simulink model "adaptive_try2"  (R2020a)
settings: Solver=VariableStepAuto  StartTime=0.0  StopTime=10.0  RelTol=1e-3
libraries: powerlib_meascontrol x6
settings Model: Creator=sulai  LastModifiedBy=sulai

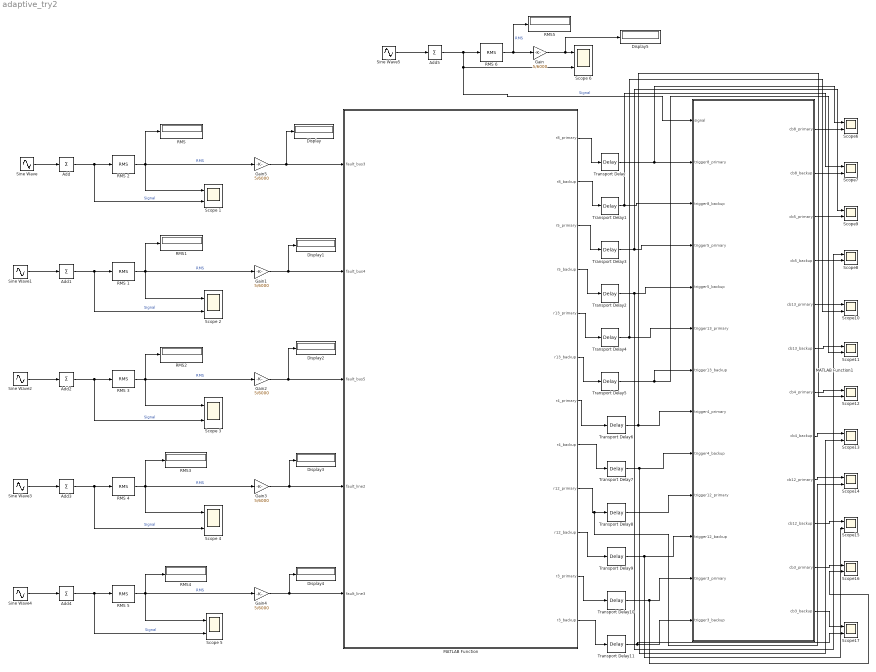
== system adaptive_try2 ==
  Add{,1..5} (6 alike) : Sum  Inputs=+  SampleTime=0
  Display{,1..5} (6 alike) : Display
  Gain{,1..5} (6 alike) : Gain  Gain=5/6000
  MATLAB Function : MATLAB Function  TreatAsAtomicUnit=on
  MATLAB Function1 : MATLAB Function  TreatAsAtomicUnit=on
  RMS{,1..5} (6 alike) : Display
      settings: Format=bank
  RMS {1..4} (4 alike) : powerlib_meascontrol/Measurements/RMS  TrueRMS=off  Freq=60  RMSInit=120  Ts=0
  RMS 5 : powerlib_meascontrol/Measurements/RMS  TrueRMS=off  Freq=10  RMSInit=120  Ts=0
  RMS 6 : powerlib_meascontrol/Measurements/RMS  TrueRMS=off  Freq=10  RMSInit=120  Ts=0
  Scope {1..6} (6 alike) : Scope  NumInputPorts=2
  Scope{6..17} (12 alike) : Scope  NumInputPorts=2
  Sine Wave{,1..3} (4 alike) : Sin  Amplitude=2  Frequency=2*pi*60  SampleTime=0
  Sine Wave4 : Sin  Amplitude=9000  Frequency=2*pi*10  SampleTime=0
  Sine Wave5 : Sin  Amplitude=126000  Frequency=2*pi*10  SampleTime=0
  Transport Delay{,3..4,6,8,10} (6 alike) : TransportDelay  DelayTime=0.2
  Transport Delay{1..2,5,7,9,11} (6 alike) : TransportDelay  DelayTime=1.86
  wires:
  MATLAB Function/2(r8_backup) -> Transport Delay1/1
  MATLAB Function/3(r5_primary) -> Transport Delay3/1
  MATLAB Function/4(r5_backup) -> Transport Delay2/1
  MATLAB Function/5(r13_primary) -> Transport Delay4/1
  MATLAB Function/6(r13_backup) -> Transport Delay5/1
  MATLAB Function/7(r4_primary) -> Transport Delay6/1
  MATLAB Function/8(r4_backup) -> Transport Delay7/1
  MATLAB Function/9(r12_primary) -> Scope14/2, Transport Delay8/1
  MATLAB Function/11(r3_primary) -> Transport Delay10/1
  MATLAB Function/12(r3_backup) -> Transport Delay11/1
  MATLAB Function/1(r8_primary) -> Transport Delay/1
  MATLAB Function/10(r12_backup) -> Transport Delay9/1
  Transport Delay9/1 -> Scope15/2, MATLAB Function1/11(trigger12_backup)
  Transport Delay8/1 -> MATLAB Function1/10(trigger12_primary)
  Transport Delay7/1 -> Scope13/2, MATLAB Function1/9(trigger4_backup)
  Transport Delay6/1 -> Scope12/2, MATLAB Function1/8(trigger4_primary)
  Transport Delay5/1 -> Scope11/2, MATLAB Function1/7(trigger13_backup)
  Transport Delay4/1 -> Scope10/2, MATLAB Function1/6(trigger13_primary)
  Transport Delay2/1 -> Scope8/1, MATLAB Function1/5(trigger5_backup)
  Transport Delay3/1 -> Scope9/1, MATLAB Function1/4(trigger5_primary)
  Transport Delay1/1 -> Scope7/1, MATLAB Function1/3(trigger8_backup)
  Transport Delay/1 -> Scope6/1, MATLAB Function1/2(trigger8_primary)
  MATLAB Function1/1(cb8_primary) -> Scope6/2
  MATLAB Function1/2(cb8_backup) -> Scope7/2
  MATLAB Function1/3(cb5_primary) -> Scope9/2
  MATLAB Function1/4(cb5_backup) -> Scope8/2
  MATLAB Function1/5(cb13_primary) -> Scope10/1
  MATLAB Function1/6(cb13_backup) -> Scope11/1
  MATLAB Function1/7(cb4_primary) -> Scope12/1
  MATLAB Function1/8(cb4_backup) -> Scope13/1
  MATLAB Function1/9(cb12_primary) -> Scope14/1
  MATLAB Function1/10(cb12_backup) -> Scope15/1
  MATLAB Function1/11(cb3_primary) -> Scope16/1
  MATLAB Function1/12(cb3_backup) -> Scope17/1
  Transport Delay10/1 -> Scope16/2, MATLAB Function1/12(trigger3_primary)
  Transport Delay11/1 -> Scope17/2, MATLAB Function1/13(trigger3_backup)
  Sine Wave/1 -> Add/1
  RMS 2/1 -> Scope 1/1, RMS/1, Gain5/1  "RMS"
  Add/1 -> Scope 1/2, RMS 2/1  "Signal"
  Gain5/1 -> Display/1, MATLAB Function/1(fault_bus3)
  Gain1/1 -> Display1/1, MATLAB Function/2(fault_bus4)
  Add1/1 -> Scope 2/2, RMS 1/1  "Signal"
  RMS 1/1 -> Scope 2/1, RMS1/1, Gain1/1  "RMS"
  Sine Wave1/1 -> Add1/1
  Gain2/1 -> Display2/1, MATLAB Function/3(fault_bus5)
  Add2/1 -> Scope 3/2, RMS 3/1  "Signal"
  RMS 3/1 -> Scope 3/1, RMS2/1, Gain2/1  "RMS"
  Sine Wave2/1 -> Add2/1
  Gain3/1 -> Display3/1, MATLAB Function/4(fault_line2)
  Add3/1 -> Scope 4/2, RMS 4/1  "Signal"
  RMS 4/1 -> Scope 4/1, RMS3/1, Gain3/1  "RMS"
  Sine Wave3/1 -> Add3/1
  Gain4/1 -> Display4/1, MATLAB Function/5(fault_line3)
  Add4/1 -> Scope 5/2, RMS 5/1  "Signal"
  RMS 5/1 -> Scope 5/1, RMS4/1, Gain4/1  "RMS"
  Sine Wave4/1 -> Add4/1
  Add5/1 -> MATLAB Function1/1(signal), Scope 6/2, RMS 6/1  "Signal"
  RMS 6/1 -> RMS5/1, Gain/1  "RMS"
  Sine Wave5/1 -> Add5/1
  Gain/1 -> Display5/1, Scope 6/1

== matlab function adaptive_try2/MATLAB Function1 ==
  data: cb8_primary output; signal input; cb8_backup output; trigger8_primary input; trigger8_backup input; trigger5_primary input; trigger5_backup input; trigger13_primary input; trigger13_backup input; trigger4_primary input; trigger4_backup input; trigger12_primary input; trigger12_backup input; trigger3_primary input; cb5_primary output; cb5_backup output; cb13_primary output; cb13_backup output; cb4_primary output; cb4_backup output; cb12_primary output; cb12_backup output; cb3_primary output; cb3_backup output; trigger3_backup input
function [cb8_primary, cb8_backup, cb5_primary, cb5_backup, cb13_primary, cb13_backup, cb4_primary, cb4_backup, cb12_primary, cb12_backup, cb3_primary, cb3_backup] = fcn(signal, trigger8_primary, trigger8_backup, trigger5_primary, trigger5_backup, trigger13_primary, trigger13_backup, trigger4_primary, trigger4_backup, trigger12_primary, trigger12_backup, trigger3_primary, trigger3_backup)

if trigger8_primary
    cb8_primary = 0;
    
else
    cb8_primary = signal;
    
end

if trigger8_backup
    cb8_backup = 0;
    
else
    cb8_backup = signal;
    
end

if trigger5_primary
    cb5_primary = 0;
    
else
    cb5_primary = signal;
    
end

if trigger5_backup
    cb5_backup = 0;
    
else
    cb5_backup = signal;
    
end

if trigger13_primary
    cb13_primary = 0;
    
else
    cb13_primary = signal;
    
end

if trigger13_backup
    cb13_backup = 0;
    
else
    cb13_backup = signal;
    
end

if trigger4_primary
    cb4_primary = 0;
    
else
    cb4_primary = signal;
    
end

if trigger4_backup
    cb4_backup = 0;
    
else
    cb4_backup = signal;
    
end

if trigger12_primary
    cb12_primary = 0;
    
else
    cb12_primary = signal;
    
end

if trigger12_backup
    cb12_backup = 0;
    
else
    cb12_backup = signal;
    
end

if trigger3_primary
    cb3_primary = 0;
    
else
    cb3_primary = signal;
    
end

if trigger3_backup
    cb3_backup = 0;
    
else
    cb3_backup = signal;
    
end

== matlab function adaptive_try2/MATLAB Function ==
  data: fault_bus3 input; r8_primary output; fault_bus4 input; fault_bus5 input; fault_line2 input; fault_line3 input; r8_backup output; r5_primary output; r5_backup output; r13_primary output; r13_backup output; r4_primary output; r4_backup output; r12_primary output; r12_backup output; r3_primary output; r3_backup output
function [r8_primary, r8_backup, r5_primary, r5_backup, r13_primary, r13_backup, r4_primary, r4_backup, r12_primary, r12_backup, r3_primary, r3_backup] = fcn(fault_bus3, fault_bus4, fault_bus5, fault_line2, fault_line3)
mode = 1;
relay_fail = 0;
I_pickup_grid = 72.87;
I_pickup_islanded = 5.13;

if mode
    if relay_fail                      % primary relays operate if true
        if fault_bus3 >= I_pickup_grid
            r8_primary = 1;
            r8_backup = 0;
            r5_primary = 0;
            r5_backup = 0;
            r13_primary = 0;
            r13_backup = 0;
            r4_primary = 0;
            r4_backup = 0;
            r12_primary = 0;
            r12_backup = 0;
            r3_primary = 0;
            r3_backup = 0;
        elseif fault_bus4 > I_pickup_grid
            r8_primary = 0;
            r8_backup = 0;
            r5_primary = 1;
            r5_backup = 0;
            r13_primary = 0;
            r13_backup = 0;
            r4_primary = 0;
            r4_backup = 0;
            r12_primary = 0;
            r12_backup = 0;
            r3_primary = 0;
            r3_backup = 0;

        elseif fault_bus5 > I_pickup_grid
            r8_primary = 0;
            r8_backup = 0;
            r5_primary = 0;
            r5_backup = 0;
            r13_primary = 1;
            r13_backup = 0;
            r4_primary = 0;
            r4_backup = 0;
            r12_primary = 0;
            r12_backup = 0;
            r3_primary = 0;
            r3_backup = 0;
            
        elseif fault_line2 > I_pickup_grid
            r8_primary = 0;
            r8_backup = 0;
            r5_primary = 0;
            r5_backup = 0;
            r13_primary = 0;
            r13_backup = 0;
            r4_primary = 1;
            r4_backup = 0;
            r12_primary = 0;
            r12_backup = 0;
            r3_primary = 0;
            r3_backup = 0;
            
        elseif fault_line3 > I_pickup_grid
            r8_primary = 0;
            r8_backup = 0;
            r5_primary = 0;
            r5_backup = 0;
            r13_primary = 0;
            r13_backup = 0;
            r4_primary = 0;
            r4_backup = 0;
            r12_primary = 1;
            r12_backup = 0;
            r3_primary = 0;
            r3_backup = 0;
            
        else
            r8_primary = 0;
            r8_backup = 0;
            r5_primary = 0;
            r5_backup = 0;
            r13_primary = 0;
            r13_backup = 0;
            r4_primary = 0;
            r4_backup = 0;
            r12_primary = 0;
            r12_backup = 0;
            r3_primary = 0;
            r3_backup = 0;
            
        end
        
    else
        if fault_bus3 > I_pickup_grid 
            r8_primary = 0;
            r8_backup = 0;
            r5_primary = 0;
            r5_backup = 0;
            r13_primary = 0;
            r13_backup = 0;
            r4_primary = 0;
            r4_backup = 1;
            r12_primary = 0;
            r12_backup = 1;
            r3_primary = 0;
            r3_backup = 1;
            
        elseif fault_bus4 > I_pickup_grid
            r8_primary = 0;
            r8_backup = 0;
            r5_primary = 0;
            r5_backup = 0;
            r13_primary = 0;
            r13_backup = 0;
            r4_primary = 0;
            r4_backup = 1;
            r12_primary = 0;
            r12_backup = 0;
            r3_primary = 0;
            r3_backup = 0;

        elseif fault_bus5 > I_pickup_grid
            r8_primary = 0;
            r8_backup = 0;
            r5_primary = 0;
            r5_backup = 1;
            r13_primary = 0;
            r13_backup = 0;
            r4_primary = 0;
            r4_backup = 1;
            r12_primary = 0;
            r12_backup = 1;
            r3_primary = 0;
            r3_backup = 0;
            
        elseif fault_line2 > I_pickup_grid
            r8_primary = 0;
            r8_backup = 1;
            r5_primary = 0;
            r5_backup = 1;
            r13_primary = 0;
            r13_backup = 0;
            r4_primary = 0;
            r4_backup = 0;
            r12_primary = 0;
            r12_backup = 1;
            r3_primary = 0;
            r3_backup = 0;
            
        elseif fault_line3 > I_pickup_grid
            r8_primary = 0;
            r8_backup = 1;
            r5_primary = 0;
            r5_backup = 0;
            r13_primary = 0;
            r13_backup = 1;
            r4_primary = 0;
            r4_backup = 1;
            r12_primary = 0;
            r12_backup = 0;
            r3_primary = 0;
            r3_backup = 0;
            
        else
            r8_primary = 0;
            r8_backup = 0;
            r5_primary = 0;
            r5_backup = 0;
            r13_primary = 0;
            r13_backup = 0;
            r4_primary = 0;
            r4_backup = 0;
            r12_primary = 0;
            r12_backup = 0;
            r3_primary = 0;
            r3_backup = 0;
            
        end
    end
else
    if relay_fail
        if fault_bus3 > I_pickup_islanded
            r8_primary = 1;
            r8_backup = 0;
            r5_primary = 0;
            r5_backup = 0;
            r13_primary = 0;
            r13_backup = 0;
            r4_primary = 0;
            r4_backup = 0;
            r12_primary = 0;
            r12_backup = 0;
            r3_primary = 0;
            r3_backup = 0;
        elseif fault_bus4 > I_pickup_islanded
            r8_primary = 0;
            r8_backup = 0;
            r5_primary = 1;
            r5_backup = 0;
            r13_primary = 0;
            r13_backup = 0;
            r4_primary = 0;
            r4_backup = 0;
            r12_primary = 0;
            r12_backup = 0;
            r3_primary = 0;
            r3_backup = 0;

        elseif fault_bus5 > I_pickup_islanded
            r8_primary = 0;
            r8_backup = 0;
            r5_primary = 0;
            r5_backup = 0;
            r13_primary = 1;
            r13_backup = 0;
            r4_primary = 0;
            r4_backup = 0;
            r12_primary = 0;
            r12_backup = 0;
            r3_primary = 0;
            r3_backup = 0;
            
        elseif fault_line2 > I_pickup_islanded
            r8_primary = 0;
            r8_backup = 0;
            r5_primary = 0;
            r5_backup = 0;
            r13_primary = 0;
            r13_backup = 0;
            r4_primary = 1;
            r4_backup = 0;
            r12_primary = 0;
            r12_backup = 0;
            r3_primary = 0;
            r3_backup = 0;
            
        elseif fault_line3 > I_pickup_islanded
            r8_primary = 0;
            r8_backup = 0;
            r5_primary = 0;
            r5_backup = 0;
            r13_primary = 0;
            r13_backup = 0;
            r4_primary = 0;
            r4_backup = 0;
            r12_primary = 1;
            r12_backup = 0;
            r3_primary = 0;
            r3_backup = 0;
            
        else
            r8_primary = 0;
            r8_backup = 0;
            r5_primary = 0;
            r5_backup = 0;
            r13_primary = 0;
            r13_backup = 0;
            r4_primary = 0;
            r4_backup = 0;
            r12_primary = 0;
            r12_backup = 0;
            r3_primary = 0;
            r3_backup = 0;
            
        end
    else
        if fault_bus3 > I_pickup_islanded 
            r8_primary = 0;
            r8_backup = 0;
            r5_primary = 0;
            r5_backup = 0;
            r13_primary = 0;
            r13_backup = 0;
            r4_primary = 0;
            r4_backup = 1;
            r12_primary = 0;
            r12_backup = 1;
            r3_primary = 0;
            r3_backup = 1;
            
        elseif fault_bus4 > I_pickup_islanded
            r8_primary = 0;
            r8_backup = 0;
            r5_primary = 0;
            r5_backup = 0;
            r13_primary = 0;
            r13_backup = 0;
            r4_primary = 0;
            r4_backup = 1;
            r12_primary = 0;
            r12_backup = 0;
            r3_primary = 0;
            r3_backup = 0;

        elseif fault_bus5 > I_pickup_islanded
            r8_primary = 0;
            r8_backup = 0;
            r5_primary = 0;
            r5_backup = 1;
            r13_primary = 0;
            r13_backup = 0;
            r4_primary = 0;
            r4_backup = 1;
            r12_primary = 0;
            r12_backup = 1;
            r3_primary = 0;
            r3_backup = 0;
            
        elseif fault_line2 > I_pickup_islanded
            r8_primary = 0;
            r8_backup = 1;
            r5_primary = 0;
            r5_backup = 1;
            r13_primary = 0;
            r13_backup = 0;
            r4_primary = 0;
            r4_backup = 0;
            r12_primary = 0;
            r12_backup = 1;
            r3_primary = 0;
            r3_backup = 0;
            
        elseif fault_line3 > I_pickup_islanded
            r8_primary = 0;
            r8_backup = 1;
            r5_primary = 0;
            r5_backup = 0;
            r13_primary = 0;
            r13_backup = 1;
            r4_primary = 0;
            r4_backup = 1;
            r12_primary = 0;
            r12_backup = 0;
            r3_primary = 0;
            r3_backup = 0;
            
        else
            r8_primary = 0;
            r8_backup = 0;
            r5_primary = 0;
            r5_backup = 0;
            r13_primary = 0;
            r13_backup = 0;
            r4_primary = 0;
            r4_backup = 0;
            r12_primary = 0;
            r12_backup = 0;
            r3_primary = 0;
            r3_backup = 0;
            
        end
    end
end
